simulink model "TBRe19_ECU_1_WORKING_190718"  (R2017b)
settings: Solver=FixedStepDiscrete  StartTime=0.0  StopTime=inf  FixedStep=0.0001  RelTol=1e-3
PostLoadFcn:
  | model_init();
libraries: simulink x17
(part 1 of 6)
settings Model: SimulationMode=external  Creator=agf25  LastModifiedBy=Peter
settings DataIOCC: LimitDataPoints=on
settings OptimizationCC: DefaultParameterBehavior=Inlined  EfficientFloat2IntCast=on  LifeSpan=inf
settings DebuggingCC: AllowSymbolicDim=off  SFUnexpectedBacktrackingDiag=warning  SFNoUnconditionalDefaultTransitionDiag=warning  SFExecutionAtInitializationDiag=none
settings ModelReferenceCC: PropagateSignalLabelsOutOfModel=off
settings RTWCC: SystemTargetFile=nsi_mpc.tlc  MakeCommand=nsi_make  TemplateMakefile=nsi_mpc.tmf  Description=RTW Coder for MUXLAB4
settings CodeAppCC: StateflowObjectComments=on
settings STFCustomTargetCC: MATLABClassNameForMDSCustomization=Simulink.SoftwareTarget.TargetSpecificTriggerConfigurationBase  SystemTargetFile=nsi_mpc.tlc
settings ConfigComp: CovMetricSettings=dw  CovHtmlReporting=on  CovSaveCumulativeToWorkspaceVar=on  CovSaveSingleToWorkspaceVar=on  CovExternalEMLEnable=off
settings SimscapeCC: SimscapeNormalizeSystem=off
settings ConfigurationSet: Description=SimMechanics 2G

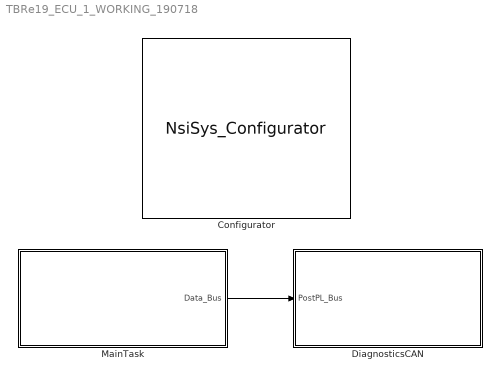
== system TBRe19_ECU_1_WORKING_190718 ==
  Configurator : S-Function  FunctionName=NsiSys_Configurator  Parameters=main,io,nbof_can,can,ccp,flash,nbof_lin,lin,tasks  SFunctionDeploymentMode=off  EnableBusSupport=off  mask(Configurator block){main=Config description;01/01/2011;0;0.000000, io=2.5;0;1;1;1;1;1;1;1, nbof_can=5, can=1;HIGH_SPEED;500Kbps;No;C:\Users\Peter\Google_Drive\Year_5\TBRe\03-Design_Files\ECU\ECU-Model\TBRe19_DBC.dbc;0;1;1Mbits;0;HIGH_SPEED;500Kbps;120 Ohm;C:\Users\TBRe-admin\Documents\Database\TBRe19_DBC_190517.dbc;0;0;1Mbits;0;HIGH_SPEED;1000Kbps;120 Ohm;D:\TOOLS\MUXLINK\R2011b\MUXlink\misc\BASE_CAN_MUXLAB4.dbc;0;0;1Mbits;0;HIGH_SPEED;500Kbps;120 Ohm;D:\TOOLS\MUXLINK\R2011b\MUXlink\misc\j1939_adapt.dbc;0;1;1Mbits;0;HIGH_SPEED;1000Kbps;No;D:\TOOLS\MUXLINK\R2011b\MUXlink\misc\BASE_CAN_MUXLAB4.dbc;0;0;1Mbits, ccp=2;0x100;0x200;0;0;0x0;0x0;0;0x13, flash=Gearing_Ratio;No;Unsigned Byte;3;1;Wheel_Size;No;Unsigned Byte;450;1;Brake1_High;No;Unsigned Word;900;1;Brake2_High;No;Unsigned Word;900;1;Throttle1_High;No;Unsigned Word;4800;1;Throttle2_High;No;Unsigned Word;4200;1;Brake1_Low;No;Unsigned Word;500;1;Brake2_Low;No;Unsigned Word;500;1;Throttle1_Low;No;Unsigned Word;904;1;Throttle2_Low;No;Unsigned Word;290;1;Max_Torque_Std;No;Unsigned Byte;140;1;Max_Torque_Boost;No;Unsigned Byte;240;1;MCU_Ignition;No;Boolean;1;1;LV_Low_Voltage_Warning;No;Unsigned Word;25000;1;MCUMotor_Temp_Warning;No;Unsigned Word;60;1;Target_Slip_Ratio;No;Single Float;0.15;1;TC_P_Gain;No;Unsigned Byte;1000;1;MinTC_Torque;No;Unsigned Byte;20;1;Max_Regen;No;Unsigned Byte;30;1;Throttle_Active_Threshold;No;Unsigned Byte;5;1;Brake_Active_Threshold;No;Unsigned Byte;15;1;INV_Torque_limit;No;Signed Word;210;1;INV_Speed_Limit_Fwd;No;Signed Word;3000;1;INV_Speed_limit_Rev;No;Signed Word;-3000;1;INV_DC_Link_Target;No;Signed Word;60;1;INV_DC_Link_Regen_Imax;No;Signed Word;-10;1;INV_DC_Link_Discharge_Imax;No;Signed Word;200;1;INV_Regen_Torque_Limit;No;Signed Word;-10;1;INV_Id_Debug;No;Signed Word;0;1;INV_Iq_debug;No;Signed Word;0;1, nbof_lin=2, lin=0;D:\TOOLS\MUXLINK\R2011b\MUXlink\misc\lindb.ldf;1;0.0;0.0;0.000;0.000;0.000000;0,0;0;D:\TOOLS\MUXLINK\R2011b\MUXlink\misc\lindb.ldf;1;0.0;0.0;0.000;0.000;0.000000;0,0, tasks=DiagnosticsCAN;[0.1];MainTask;[0.01]}
      mask prompts: nbof_can "nbof can"
      mask help: This block permits to set general parameters to use a MUXlink model
      mask init:
      | NsiSys_Configurator_InitializationFcn();
      settings: OpenFcn=NsiSys_Configurator_OpenFcn();
      mask Help:
      | eval('block=get_param(gcb, ''RTWdata'');')
      | web([docroot '\toolbox\MUXlink\html\blocks/' block.MUXlink_BlockType '.html'])
      mask Callback main: NsiSys_Configurator_ApplyFcn(1);
      mask Callback io: NsiSys_Configurator_ApplyFcn(2);
      mask Callback nbof_can: NsiSys_Configurator_ApplyFcn(3);
      mask Callback can: NsiSys_Configurator_ApplyFcn(4);
      mask Callback ccp: NsiSys_Configurator_ApplyFcn(5);
      mask Callback flash: NsiSys_Configurator_ApplyFcn(6);
      mask Callback nbof_lin: NsiSys_Configurator_ApplyFcn(7);
      mask Callback lin: NsiSys_Configurator_ApplyFcn(8);
      mask Callback tasks: NsiSys_Configurator_ApplyFcn(9);
      mask Display: image(imread('MUXLAB4.bmp'));text(0.5, 0.2, '', 'horizontalAlignment', 'center', 'verticalAlignment', 'base');
  DiagnosticsCAN : Subsystem  TreatAsAtomicUnit=on  SystemSampleTime=[0.1]  RTWFcnName=DiagnosticsCAN  RTWFileName=FileTaskFcn
      mask init:
      | NsiSys_SubSystemTask_InitializationFcn();
      settings: OpenFcn=NsiSys_SubSystemTask_OpenFcn();  RTWSystemCode=Nonreusable function  RTWFcnNameOpts=User specified  RTWFileNameOpts=Use function name
      mask Display: image(imread('nsi.bmp'));text(0.45, 0.9, 'task()');plot([0.05 0.05 0.05 0.05 0.05 0.05 0.05 0.05 0.05 0.05]);fprintf('DiagnosticsCAN\n/ 100.0ms / 10.0ms /\nEvent');
  MainTask : Subsystem  TreatAsAtomicUnit=on  SystemSampleTime=[0.01]  RTWFcnName=MainTask  RTWFileName=FileTaskFcn
      mask init:
      | NsiSys_SubSystemTask_InitializationFcn();
      settings: OpenFcn=NsiSys_SubSystemTask_OpenFcn();  RTWSystemCode=Nonreusable function  RTWFcnNameOpts=User specified  RTWFileNameOpts=Use function name
      mask Display: image(imread('nsi.bmp'));text(0.45, 0.9, 'task()');plot([0.05 0.05 0.05 0.05 0.05 0.05 0.05 0.05 0.05 0.05]);fprintf('MainTask\n/ 10.0ms / 0.0ms /\nEvent');
  wires:
  MainTask/1(Data_Bus) -> DiagnosticsCAN/1(PostPL_Bus)

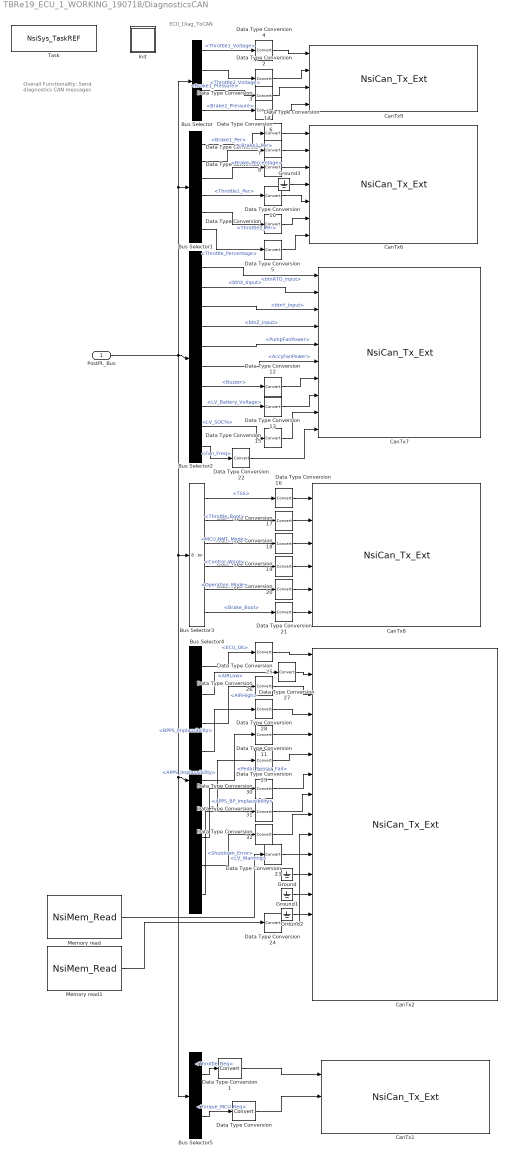
== system TBRe19_ECU_1_WORKING_190718/DiagnosticsCAN ==
  note: ECU_Diag_ToCAN
  note: Overall Functionality:
      | Send diagnostics CAN messages
  PostPL_Bus : Inport
  Bus Selector : BusSelector  OutputSignals=VFL_Data.PrePL_Data.DAL_Data.DAL_Hardwired.Throttle1_Voltage,VFL_Data.PrePL_Data.DAL_Data.DAL_Hardwired.Throttle2_Voltage,VFL_Data.PrePL_Data.DAL_Data.DAL_Hardwired.Brake1_Pressure,VFL_Data.PrePL_Data.DAL_Data.DAL_Hardwired.Brake2_Pressure
  Bus Selector1 : BusSelector  OutputSignals=VFL_Data.PrePL_Data.Pedal_Box_Data.Brake1_Per,VFL_Data.PrePL_Data.Pedal_Box_Data.Brake2_Per,VFL_Data.PrePL_Data.Pedal_Box_Data.Brake_Percentage,VFL_Data.PrePL_Data.Pedal_Box_Data.Throttle1_Per,VFL_Data.PrePL_Data.Pedal_Box_Data.Throttle2_Per,VFL_Data.PrePL_Data.Pedal_Box_Data.Throttle_Percentage
  Bus Selector2 : BusSelector  OutputSignals=VFL_Data.PrePL_Data.DAL_Data.DAL_Hardwired.btnRTD_Input,VFL_Data.PrePL_Data.DAL_Data.DAL_Hardwired.btnX_Input,VFL_Data.PrePL_Data.DAL_Data.DAL_Hardwired.btnY_Input,VFL_Data.PrePL_Data.DAL_Data.DAL_Hardwired.btnZ_Input,Hardwired_Peripherals.PumpFanPower,Hardwired_Peripherals.AccyFanPower,Hardwired_Peripherals.Buzzer,VFL_Data.PrePL_Data.LV_Battery.LV_Battery_Voltage,VFL_Data.PrePL_Data.LV_Battery.LV_SOC%,VFL_Data.PrePL_Data.DAL_Data.DAL_Hardwired.Fan_Freq
  Bus Selector3 : BusSelector  OutputSignals=VFL_Data.VOM_Data.TSS,VFL_Data.PrePL_Data.Pedal_Box_Data.Throttle_Bool,VFL_Data.VOM_Data.MCU_NMT_Mode,VFL_Data.VOM_Data.Control_Word,VFL_Data.VOM_Data.Operation_Mode,VFL_Data.PrePL_Data.Pedal_Box_Data.Brake_Bool
  Bus Selector4 : BusSelector  OutputSignals=Hardwired_Peripherals.ECU_Ok,VFL_Data.PrePL_Data.DAL_Data.DAL_Hardwired.AIRLow,VFL_Data.PrePL_Data.DAL_Data.DAL_Hardwired.AIRHigh,VFL_Data.PrePL_Data.Pedal_Box_Data.BPPS_Implausibility,VFL_Data.PrePL_Data.Pedal_Box_Data.Pedal_Sensor_Fail,VFL_Data.PrePL_Data.Pedal_Box_Data.APPS_Implausibility,VFL_Data.PrePL_Data.Pedal_Box_Data.APPS_BP_Implausibility,VFL_Data.PrePL_Data.LV_Battery.LV_Warning,VFL_Data.PrePL_Data.DAL_Data.DAL_CAN.DAL_SENSORCAN.Shutdown_Error
  Bus Selector5 : BusSelector  OutputSignals=VFL_Data.Drive_Data.Throttle_Req,VFL_Data.Drive_Data.Torque_MCU_Req
  CanTx1 : S-Function  FunctionName=NsiCan_Tx_Ext  Parameters=data_can,channel,msg_name,ident,ident_type,dlc,signals,is_physical,is_canfd,is_crc  SFunctionDeploymentMode=off  EnableBusSupport=off  mask(MUXlink Can Tx){data_can=1;HIGH_SPEED;500Kbps;No;C:\Users\TBRe-admin\Documents\TBReVCU\TBRe19_DBC.dbc;0;;;0;HIGH_SPEED;500Kbps;120 Ohm;C:\Users\TBRe-admin\Documents\Database\TBRe19_DBC_190517.dbc;0;;;0;HIGH_SPEED;1000Kbps;120 Ohm;D:\TOOLS\MUXLINK\R2011b\MUXlink\misc\BASE_CAN_MUXLAB4.dbc;0;;;0;HIGH_SPEED;500Kbps;120 Ohm;D:\TOOLS\MUXLINK\R2011b\MUXlink\misc\j1939_adapt.dbc;0;;;0;HIGH_SPEED;1000Kbps;No;D:\TOOLS\MUXLINK\R2011b\MUXlink\misc\BASE_CAN_MUXLAB4.dbc;0;;, channel=1, msg_name=VCU_Torque, ident=0x706, ident_type=STD, dlc=5, signals=ECU_TorqueReq;1;0;-16;0.100000;0.000000;Percent;ECU_TorqueAcut;1;16;-16;0.100000;0.000000;Percent;Max_Torque;1;32;-8;1.000000;0.000000;_, is_physical=1, is_canfd=0, is_crc=0}
      mask prompts: data_can "data can"; msg_name "msg name"
      mask help: Transmit a frame on a CAN Channel.
      mask init:
      | NsiCan_Tx_Ext_InitializationFcn();
      settings: OpenFcn=NsiCan_Tx_Ext_OpenFcn();
      mask Help:
      | eval('block=get_param(gcb, ''RTWdata'');')
      | web([docroot '\toolbox\MUXlink\html\blocks/' block.MUXlink_BlockType '.html'])
      mask Callback data_can: NsiCan_Tx_Ext_ApplyFcn(1);
      mask Callback channel: NsiCan_Tx_Ext_ApplyFcn(2);
      mask Callback msg_name: NsiCan_Tx_Ext_ApplyFcn(3);
      mask Callback ident: NsiCan_Tx_Ext_ApplyFcn(4);
      mask Callback ident_type: NsiCan_Tx_Ext_ApplyFcn(5);
      mask Callback dlc: NsiCan_Tx_Ext_ApplyFcn(6);
      mask Callback signals: NsiCan_Tx_Ext_ApplyFcn(7);
      mask Callback is_physical: NsiCan_Tx_Ext_ApplyFcn(7);
      mask Callback is_canfd: NsiCan_Tx_Ext_ApplyFcn(7);
      mask Callback is_crc: NsiCan_Tx_Ext_ApplyFcn(7);
      mask Display: image(imread('nsi.bmp'));text(0.5, 0.1, 'TX_VCU_Torque_CAN1', 'horizontalAlignment', 'center', 'verticalAlignment', 'base');plot([0.05 0.05 0.05 0.05 0.05 0.05 0.05 0.05 0.05 0.05]); port_label('input',1, 'ECU_TorqueReq'); port_label('input',2, 'ECU_TorqueAcut'); port_label('input',3, 'Max_Torque');
  CanTx2 : S-Function  FunctionName=NsiCan_Tx_Ext  Parameters=data_can,channel,msg_name,ident,ident_type,dlc,signals,is_physical,is_canfd,is_crc  SFunctionDeploymentMode=off  EnableBusSupport=off  mask(MUXlink Can Tx){data_can=1;HIGH_SPEED;500Kbps;No;C:\Users\TBRe-admin\Documents\TBReVCU\TBRe19_DBC.dbc;0;;;0;HIGH_SPEED;500Kbps;120 Ohm;C:\Users\TBRe-admin\Documents\Database\TBRe19_DBC_190517.dbc;0;;;0;HIGH_SPEED;1000Kbps;120 Ohm;D:\TOOLS\MUXLINK\R2011b\MUXlink\misc\BASE_CAN_MUXLAB4.dbc;0;;;0;HIGH_SPEED;500Kbps;120 Ohm;D:\TOOLS\MUXLINK\R2011b\MUXlink\misc\j1939_adapt.dbc;0;;;0;HIGH_SPEED;1000Kbps;No;D:\TOOLS\MUXLINK\R2011b\MUXlink\misc\BASE_CAN_MUXLAB4.dbc;0;;, channel=1, msg_name=VCU_Diagnostics, ident=0x700, ident_type=STD, dlc=4, signals=Shutdown_ECU;1;22;-1;1.000000;0.000000;_;Low_AIR_Status;1;20;-1;1.000000;0.000000;_;High_AIR_Status;1;21;1;1.000000;0.000000;_;BPPS_Implausibility;1;16;-1;1.000000;0.000000;_;Pedal_Sensor_Fail;1;24;8;1.000000;0.000000;_;APPS_Implausibility;1;17;1;1.000000;0.000000;_;APPS_BP_Implausibility;1;18;1;1.000000;0.000000;_;Shutdown_CarShutdown;1;23;1;1.000000;0.000000;_;LV_Battery_Warning;1;19;1;1.000000;0.000000;_;GearingRatio;1;8;8;0.100000;0.000000;_;Wheel_Size;1;0;8;0.100000;0.000000;m;Boost_on;1;34;-1;1.000000;0.000000;_;TC_on;1;33;-1;1.000000;0.000000;_;RegenBool;1;32;-1;1.000000;0.000000;_;VCU_Day;1;35;5;1.000000;0.000000;_;VCU_Month;1;40;8;1.000000;0.000000;_;VCU_Version;1;56;8;1.000000;0.000000;_;VCU_Year;1;48;8;1.000000;0.000000;_, is_physical=1, is_canfd=0, is_crc=0}
      mask prompts: data_can "data can"; msg_name "msg name"
      mask help: Transmit a frame on a CAN Channel.
      mask init:
      | NsiCan_Tx_Ext_InitializationFcn();
      settings: OpenFcn=NsiCan_Tx_Ext_OpenFcn();
      mask Help:
      | eval('block=get_param(gcb, ''RTWdata'');')
      | web([docroot '\toolbox\MUXlink\html\blocks/' block.MUXlink_BlockType '.html'])
      mask Callback data_can: NsiCan_Tx_Ext_ApplyFcn(1);
      mask Callback channel: NsiCan_Tx_Ext_ApplyFcn(2);
      mask Callback msg_name: NsiCan_Tx_Ext_ApplyFcn(3);
      mask Callback ident: NsiCan_Tx_Ext_ApplyFcn(4);
      mask Callback ident_type: NsiCan_Tx_Ext_ApplyFcn(5);
      mask Callback dlc: NsiCan_Tx_Ext_ApplyFcn(6);
      mask Callback signals: NsiCan_Tx_Ext_ApplyFcn(7);
      mask Callback is_physical: NsiCan_Tx_Ext_ApplyFcn(7);
      mask Callback is_canfd: NsiCan_Tx_Ext_ApplyFcn(7);
      mask Callback is_crc: NsiCan_Tx_Ext_ApplyFcn(7);
      mask Display: image(imread('nsi.bmp'));text(0.5, 0.3, 'TX_VCU_Diagnostics_CAN1', 'horizontalAlignment', 'center', 'verticalAlignment', 'base');plot([0.05 0.05 0.05 0.05 0.05 0.05 0.05 0.05 0.05 0.05]); port_label('input',1, 'Shutdown_ECU'); port_label('input',2, 'Low_AIR_Status'); port_label('input',3, 'High_AIR_Status'); port_label('input',4, 'BPPS_Implausibility'); port_label('input',5, 'Pedal_Sensor_Fail'); port_label('input',6, 'APPS_Implausibility'); port_label('input',7, 'APPS_BP_Implausibility'); port_label('input',8, 'Shutdown_CarShutdown'); port_label('input',9, 'LV_Battery_Warning'); port_label('input',10, 'GearingRatio'); port_label('input',11, 'Wheel_Size'); port_label('input',12, 'Boost_on'); port_label('input',13, 'TC_on'); port_label('input',14, 'RegenBool'); port_label('input',15, 'VCU_Day'); port_label('input',16, 'VCU_Month'); port_label('input',17, 'VCU_Version'); port_label('input',18, 'VCU_Year');
  CanTx6 : S-Function  FunctionName=NsiCan_Tx_Ext  Parameters=data_can,channel,msg_name,ident,ident_type,dlc,signals,is_physical,is_canfd,is_crc  SFunctionDeploymentMode=off  EnableBusSupport=off  mask(MUXlink Can Tx){data_can=1;HIGH_SPEED;500Kbps;No;C:\Users\TBRe-admin\Documents\TBReVCU\TBRe19_DBC.dbc;0;;;0;HIGH_SPEED;500Kbps;120 Ohm;C:\Users\TBRe-admin\Documents\Database\TBRe19_DBC_190517.dbc;0;;;0;HIGH_SPEED;1000Kbps;120 Ohm;D:\TOOLS\MUXLINK\R2011b\MUXlink\misc\BASE_CAN_MUXLAB4.dbc;0;;;0;HIGH_SPEED;500Kbps;120 Ohm;D:\TOOLS\MUXLINK\R2011b\MUXlink\misc\j1939_adapt.dbc;0;;;0;HIGH_SPEED;1000Kbps;No;D:\TOOLS\MUXLINK\R2011b\MUXlink\misc\BASE_CAN_MUXLAB4.dbc;0;;, channel=1, msg_name=VCU_Pedal_Percentages, ident=0x702, ident_type=STD, dlc=7, signals=Brake1_Percentage;1;24;8;1.000000;0.000000;%;Brake2_Percentage;1;32;8;1.000000;0.000000;%;Brake_Percentage;1;48;8;1.000000;0.000000;%;BrakePot_Percentage;1;40;8;1.000000;0.000000;%;Throttle1_Percent;1;0;8;1.000000;0.000000;%;Throttle2_Percentage;1;8;8;1.000000;0.000000;%;Throttle_Percentage;1;16;8;1.000000;0.000000;%, is_physical=1, is_canfd=0, is_crc=0}
      mask prompts: data_can "data can"; msg_name "msg name"
      mask help: Transmit a frame on a CAN Channel.
      mask init:
      | NsiCan_Tx_Ext_InitializationFcn();
      settings: OpenFcn=NsiCan_Tx_Ext_OpenFcn();
      mask Help:
      | eval('block=get_param(gcb, ''RTWdata'');')
      | web([docroot '\toolbox\MUXlink\html\blocks/' block.MUXlink_BlockType '.html'])
      mask Callback data_can: NsiCan_Tx_Ext_ApplyFcn(1);
      mask Callback channel: NsiCan_Tx_Ext_ApplyFcn(2);
      mask Callback msg_name: NsiCan_Tx_Ext_ApplyFcn(3);
      mask Callback ident: NsiCan_Tx_Ext_ApplyFcn(4);
      mask Callback ident_type: NsiCan_Tx_Ext_ApplyFcn(5);
      mask Callback dlc: NsiCan_Tx_Ext_ApplyFcn(6);
      mask Callback signals: NsiCan_Tx_Ext_ApplyFcn(7);
      mask Callback is_physical: NsiCan_Tx_Ext_ApplyFcn(7);
      mask Callback is_canfd: NsiCan_Tx_Ext_ApplyFcn(7);
      mask Callback is_crc: NsiCan_Tx_Ext_ApplyFcn(7);
      mask Display: image(imread('nsi.bmp'));text(0.5, 0.1, 'TX_VCU_Pedal_Percentages_CAN1', 'horizontalAlignment', 'center', 'verticalAlignment', 'base');plot([0.05 0.05 0.05 0.05 0.05 0.05 0.05 0.05 0.05 0.05]); port_label('input',1, 'Brake1_Percentage'); port_label('input',2, 'Brake2_Percentage'); port_label('input',3, 'Brake_Percentage'); port_label('input',4, 'BrakePot_Percentage'); port_label('input',5, 'Throttle1_Percent'); port_label('input',6, 'Throttle2_Percentage'); port_label('input',7, 'Throttle_Percentage');
  CanTx7 : S-Function  FunctionName=NsiCan_Tx_Ext  Parameters=data_can,channel,msg_name,ident,ident_type,dlc,signals,is_physical,is_canfd,is_crc  SFunctionDeploymentMode=off  EnableBusSupport=off  mask(MUXlink Can Tx){data_can=1;HIGH_SPEED;500Kbps;No;C:\Users\TBRe-admin\Documents\TBReVCU\TBRe19_DBC.dbc;0;;;0;HIGH_SPEED;500Kbps;120 Ohm;C:\Users\TBRe-admin\Documents\Database\TBRe19_DBC_190517.dbc;0;;;0;HIGH_SPEED;1000Kbps;120 Ohm;D:\TOOLS\MUXLINK\R2011b\MUXlink\misc\BASE_CAN_MUXLAB4.dbc;0;;;0;HIGH_SPEED;500Kbps;120 Ohm;D:\TOOLS\MUXLINK\R2011b\MUXlink\misc\j1939_adapt.dbc;0;;;0;HIGH_SPEED;1000Kbps;No;D:\TOOLS\MUXLINK\R2011b\MUXlink\misc\BASE_CAN_MUXLAB4.dbc;0;;, channel=1, msg_name=VCU_HW_IO, ident=0x701, ident_type=STD, dlc=4, signals=Console_RTD;1;0;1;1.000000;0.000000;Bool;Console_X;1;3;1;1.000000;0.000000;Bool;Consle_Y;1;2;-1;1.000000;0.000000;Bool;Console_Z;1;1;-1;1.000000;0.000000;_;Coolant_Pump_Fan;1;5;1;1.000000;0.000000;_;Coolant_AccyFan;1;6;-1;1.000000;0.000000;_;Buzzer;1;7;1;1.000000;0.000000;_;LV_Battery_Voltage;1;16;16;1.000000;0.000000;mV;LV_Battery_SOC;1;8;8;1.000000;0.000000;_;AccyFanFreq;1;32;8;1.000000;0.000000;Hz, is_physical=1, is_canfd=0, is_crc=0}
      mask prompts: data_can "data can"; msg_name "msg name"
      mask help: Transmit a frame on a CAN Channel.
      mask init:
      | NsiCan_Tx_Ext_InitializationFcn();
      settings: OpenFcn=NsiCan_Tx_Ext_OpenFcn();
      mask Help:
      | eval('block=get_param(gcb, ''RTWdata'');')
      | web([docroot '\toolbox\MUXlink\html\blocks/' block.MUXlink_BlockType '.html'])
      mask Callback data_can: NsiCan_Tx_Ext_ApplyFcn(1);
      mask Callback channel: NsiCan_Tx_Ext_ApplyFcn(2);
      mask Callback msg_name: NsiCan_Tx_Ext_ApplyFcn(3);
      mask Callback ident: NsiCan_Tx_Ext_ApplyFcn(4);
      mask Callback ident_type: NsiCan_Tx_Ext_ApplyFcn(5);
      mask Callback dlc: NsiCan_Tx_Ext_ApplyFcn(6);
      mask Callback signals: NsiCan_Tx_Ext_ApplyFcn(7);
      mask Callback is_physical: NsiCan_Tx_Ext_ApplyFcn(7);
      mask Callback is_canfd: NsiCan_Tx_Ext_ApplyFcn(7);
      mask Callback is_crc: NsiCan_Tx_Ext_ApplyFcn(7);
      mask Display: image(imread('nsi.bmp'));text(0.5, 0.3, 'TX_VCU_HW_IO_CAN1', 'horizontalAlignment', 'center', 'verticalAlignment', 'base');plot([0.05 0.05 0.05 0.05 0.05 0.05 0.05 0.05 0.05 0.05]); port_label('input',1, 'Console_RTD'); port_label('input',2, 'Console_X'); port_label('input',3, 'Consle_Y'); port_label('input',4, 'Console_Z'); port_label('input',5, 'Coolant_Pump_Fan'); port_label('input',6, 'Coolant_AccyFan'); port_label('input',7, 'Buzzer'); port_label('input',8, 'LV_Battery_Voltage'); port_label('input',9, 'LV_Battery_SOC'); port_label('input',10, 'AccyFanFreq');
  CanTx8 : S-Function  FunctionName=NsiCan_Tx_Ext  Parameters=data_can,channel,msg_name,ident,ident_type,dlc,signals,is_physical,is_canfd,is_crc  SFunctionDeploymentMode=off  EnableBusSupport=off  mask(MUXlink Can Tx){data_can=1;HIGH_SPEED;500Kbps;No;C:\Users\TBRe-admin\Documents\TBReVCU\TBRe19_DBC.dbc;0;;;0;HIGH_SPEED;500Kbps;120 Ohm;C:\Users\TBRe-admin\Documents\Database\TBRe19_DBC_190517.dbc;0;;;0;HIGH_SPEED;1000Kbps;120 Ohm;D:\TOOLS\MUXLINK\R2011b\MUXlink\misc\BASE_CAN_MUXLAB4.dbc;0;;;0;HIGH_SPEED;500Kbps;120 Ohm;D:\TOOLS\MUXLINK\R2011b\MUXlink\misc\j1939_adapt.dbc;0;;;0;HIGH_SPEED;1000Kbps;No;D:\TOOLS\MUXLINK\R2011b\MUXlink\misc\BASE_CAN_MUXLAB4.dbc;0;;, channel=1, msg_name=VCU_Vehicle_Functionality, ident=0x704, ident_type=STD, dlc=4, signals=Tractive_System_Startup;1;24;1;1.000000;0.000000;_;Throttle_Bool;1;25;1;1.000000;0.000000;_;MCU_NMT_Mode;1;16;8;1.000000;0.000000;_;Control_Word;1;0;8;1.000000;0.000000;_;Vehicle_Operation;1;8;8;1.000000;0.000000;_;Brake_Bool;1;26;1;1.000000;0.000000;_, is_physical=1, is_canfd=0, is_crc=0}
      mask prompts: data_can "data can"; msg_name "msg name"
      mask help: Transmit a frame on a CAN Channel.
      mask init:
      | NsiCan_Tx_Ext_InitializationFcn();
      settings: OpenFcn=NsiCan_Tx_Ext_OpenFcn();
      mask Help:
      | eval('block=get_param(gcb, ''RTWdata'');')
      | web([docroot '\toolbox\MUXlink\html\blocks/' block.MUXlink_BlockType '.html'])
      mask Callback data_can: NsiCan_Tx_Ext_ApplyFcn(1);
      mask Callback channel: NsiCan_Tx_Ext_ApplyFcn(2);
      mask Callback msg_name: NsiCan_Tx_Ext_ApplyFcn(3);
      mask Callback ident: NsiCan_Tx_Ext_ApplyFcn(4);
      mask Callback ident_type: NsiCan_Tx_Ext_ApplyFcn(5);
      mask Callback dlc: NsiCan_Tx_Ext_ApplyFcn(6);
      mask Callback signals: NsiCan_Tx_Ext_ApplyFcn(7);
      mask Callback is_physical: NsiCan_Tx_Ext_ApplyFcn(7);
      mask Callback is_canfd: NsiCan_Tx_Ext_ApplyFcn(7);
      mask Callback is_crc: NsiCan_Tx_Ext_ApplyFcn(7);
      mask Display: image(imread('nsi.bmp'));text(0.5, 0.3, 'TX_VCU_Vehicle_Functionality_CAN1', 'horizontalAlignment', 'center', 'verticalAlignment', 'base');plot([0.05 0.05 0.05 0.05 0.05 0.05 0.05 0.05 0.05 0.05]); port_label('input',1, 'Tractive_System_Startup'); port_label('input',2, 'Throttle_Bool'); port_label('input',3, 'MCU_NMT_Mode'); port_label('input',4, 'Control_Word'); port_label('input',5, 'Vehicle_Operation'); port_label('input',6, 'Brake_Bool');
  CanTx9 : S-Function  FunctionName=NsiCan_Tx_Ext  Parameters=data_can,channel,msg_name,ident,ident_type,dlc,signals,is_physical,is_canfd,is_crc  SFunctionDeploymentMode=off  EnableBusSupport=off  mask(MUXlink Can Tx){data_can=1;HIGH_SPEED;500Kbps;No;C:\Users\TBRe-admin\Documents\Database\TBRe19_DBC_190621.dbc;0;;;0;HIGH_SPEED;500Kbps;120 Ohm;C:\Users\TBRe-admin\Documents\Database\TBRe19_DBC_190517.dbc;0;;;0;HIGH_SPEED;1000Kbps;120 Ohm;D:\TOOLS\MUXLINK\R2011b\MUXlink\misc\BASE_CAN_MUXLAB4.dbc;0;;;0;HIGH_SPEED;500Kbps;120 Ohm;D:\TOOLS\MUXLINK\R2011b\MUXlink\misc\j1939_adapt.dbc;0;;;0;HIGH_SPEED;1000Kbps;No;D:\TOOLS\MUXLINK\R2011b\MUXlink\misc\BASE_CAN_MUXLAB4.dbc;0;;, channel=1, msg_name=VCU_Pedal_Voltages, ident=0x703, ident_type=STD, dlc=8, signals=Throttle1_Voltage;1;0;16;1.000000;0.000000;mV;Throttle2_Voltage;1;32;16;1.000000;0.000000;mV;Brake1_Voltage;1;16;16;1.000000;0.000000;mV;Brake2_Voltage;1;48;16;1.000000;0.000000;mV, is_physical=0, is_canfd=0, is_crc=0}
      mask prompts: data_can "data can"; msg_name "msg name"
      mask help: Transmit a frame on a CAN Channel.
      mask init:
      | NsiCan_Tx_Ext_InitializationFcn();
      settings: OpenFcn=NsiCan_Tx_Ext_OpenFcn();
      mask Help:
      | eval('block=get_param(gcb, ''RTWdata'');')
      | web([docroot '\toolbox\MUXlink\html\blocks/' block.MUXlink_BlockType '.html'])
      mask Callback data_can: NsiCan_Tx_Ext_ApplyFcn(1);
      mask Callback channel: NsiCan_Tx_Ext_ApplyFcn(2);
      mask Callback msg_name: NsiCan_Tx_Ext_ApplyFcn(3);
      mask Callback ident: NsiCan_Tx_Ext_ApplyFcn(4);
      mask Callback ident_type: NsiCan_Tx_Ext_ApplyFcn(5);
      mask Callback dlc: NsiCan_Tx_Ext_ApplyFcn(6);
      mask Callback signals: NsiCan_Tx_Ext_ApplyFcn(7);
      mask Callback is_physical: NsiCan_Tx_Ext_ApplyFcn(7);
      mask Callback is_canfd: NsiCan_Tx_Ext_ApplyFcn(7);
      mask Callback is_crc: NsiCan_Tx_Ext_ApplyFcn(7);
      mask Display: image(imread('nsi.bmp'));text(0.5, 0.3, 'TX_VCU_Pedal_Voltages_CAN1', 'horizontalAlignment', 'center', 'verticalAlignment', 'base');plot([0.05 0.05 0.05 0.05 0.05 0.05 0.05 0.05 0.05 0.05]); port_label('input',1, 'Throttle1_Voltage'); port_label('input',2, 'Throttle2_Voltage'); port_label('input',3, 'Brake1_Voltage'); port_label('input',4, 'Brake2_Voltage');
  Data Type Conversion{,1..32} (33 alike) : DataTypeConversion
  Ground{,1..3} (4 alike) : Ground
  Init : Subsystem  mask(System Initialize){}
      mask help: Add code to a systems Initialize function
      settings: CopyFcn=cccopyfcn(gcb)  OpenFcn=ccopenfcn('System Initialize Function')
      mask Help: This block contains text fields to insert custom user code sections at the declaration, execution and exit sections of the systems initialize function.  By placing this block inside a subsytem, the custom user code will appear in that subsystems function.
      mask Display: disp('I()')
  Memory read : S-Function  FunctionName=NsiMem_Read  Parameters=name_var,type_var,size_var,tunable_var  SFunctionDeploymentMode=off  EnableBusSupport=off  mask(Memory read){name_var=Wheel_Size, type_var=Unsigned Byte, size_var=1, tunable_var=on}
      mask prompts: name_var "Variable name :"; type_var "Type :"; size_var "Dim of table :"; tunable_var "Is Tunable By USB?"
      mask help: Reads current value of variable memory declared in the configurator block in calibration page.
      mask init:
      | NsiMem_Read_InitializationFcn();
      settings: OpenFcn=NsiMem_Read_OpenFcn();
      mask Help:
      | eval('block=get_param(gcb, ''RTWdata'');')
      | web([docroot '\toolbox\MUXlink\html\blocks/' block.MUXlink_BlockType '.html'])
      mask TypeOptions name_var: Gearing_Ratio | Wheel_Size | Brake1_High | Brake2_High | Throttle1_High | Throttle2_High | Brake1_Low | Brake2_Low | Throttle1_Low | Throttle2_Low | Max_Torque_Std | Max_Torque_Boost | MCU_Ignition | LV_Low_Voltage_Warning | MCUMotor_Temp_Warning | Target_Slip_Ratio | TC_P_Gain | MinTC_Torque | Max_Regen | Throttle_Active_Threshold | Brake_Active_Threshold | INV_Torque_limit | INV_Speed_Limit_Fwd | INV_Speed_limit_Rev | INV_DC_Link_Target | INV_DC_Link_Regen_Imax | INV_DC_Link_Discharge_Imax | INV_Regen_Torque_Limit | INV_Id_Debug | INV_Iq_debug
      mask Callback name_var: NsiMem_Read_ApplyFcn(1);
      mask TypeOptions type_var: Boolean | Signed Byte | Unsigned Byte | Signed Word | Unsigned Word | Signed Double Word | Unsigned Double Word | Single Float | Double Float
      mask Callback type_var: NsiMem_Read_ApplyFcn(2);
      mask Callback size_var: NsiMem_Read_ApplyFcn(3);
      mask Callback tunable_var: NsiMem_Read_ApplyFcn(4);
      mask Display: image(imread('nsi.bmp'));text(0.5, 0.35, 'Wheel_Size', 'horizontalAlignment', 'center', 'verticalAlignment', 'base');plot([0.05 0.05 0.05 0.05 0.05 0.05 0.05 0.05 0.05 0.05]);port_label('output', 1, 'Read');
  Memory read1 : S-Function  FunctionName=NsiMem_Read  Parameters=name_var,type_var,size_var,tunable_var  SFunctionDeploymentMode=off  EnableBusSupport=off  mask(Memory read){name_var=Gearing_Ratio, type_var=Unsigned Byte, size_var=1, tunable_var=on}
      mask prompts: name_var "Variable name :"; type_var "Type :"; size_var "Dim of table :"; tunable_var "Is Tunable By USB?"
      mask help: Reads current value of variable memory declared in the configurator block in calibration page.
      mask init:
      | NsiMem_Read_InitializationFcn();
      settings: OpenFcn=NsiMem_Read_OpenFcn();
      mask Help:
      | eval('block=get_param(gcb, ''RTWdata'');')
      | web([docroot '\toolbox\MUXlink\html\blocks/' block.MUXlink_BlockType '.html'])
      mask TypeOptions name_var: Gearing_Ratio | Wheel_Size | Brake1_High | Brake2_High | Throttle1_High | Throttle2_High | Brake1_Low | Brake2_Low | Throttle1_Low | Throttle2_Low | Max_Torque_Std | Max_Torque_Boost | MCU_Ignition | LV_Low_Voltage_Warning | MCUMotor_Temp_Warning | Target_Slip_Ratio | TC_P_Gain | MinTC_Torque | Max_Regen | Throttle_Active_Threshold | Brake_Active_Threshold | INV_Torque_limit | INV_Speed_Limit_Fwd | INV_Speed_limit_Rev | INV_DC_Link_Target | INV_DC_Link_Regen_Imax | INV_DC_Link_Discharge_Imax | INV_Regen_Torque_Limit | INV_Id_Debug | INV_Iq_debug
      mask Callback name_var: NsiMem_Read_ApplyFcn(1);
      mask TypeOptions type_var: Boolean | Signed Byte | Unsigned Byte | Signed Word | Unsigned Word | Signed Double Word | Unsigned Double Word | Single Float | Double Float
      mask Callback type_var: NsiMem_Read_ApplyFcn(2);
      mask Callback size_var: NsiMem_Read_ApplyFcn(3);
      mask Callback tunable_var: NsiMem_Read_ApplyFcn(4);
      mask Display: image(imread('nsi.bmp'));text(0.5, 0.35, 'Gearing_Ratio', 'horizontalAlignment', 'center', 'verticalAlignment', 'base');plot([0.05 0.05 0.05 0.05 0.05 0.05 0.05 0.05 0.05 0.05]);port_label('output', 1, 'Read');
  Task : S-Function  FunctionName=NsiSys_TaskREF  Parameters=task_initialised,task_periodic, task_sampletime,task_name,task_event,task_offset  SFunctionDeploymentMode=off  EnableBusSupport=off  mask(task definition){task_initialised=on, task_periodic=on, task_sampletime=[0.1], task_offset=0.01, task_name=DiagnosticsCAN, task_event=on}
      mask prompts: task_initialised "task initialised"; task_periodic "Is Periodic"; task_sampletime "Task sample time"; task_offset "Task Offset"; task_name "Task name"; task_event "Is event"
      mask help:
      | Permit to provide all parameters associated to a MUXLINK task.
      | Task can be executed periodicaly and/or on event detection.
      | If task is periodic:
      | Task sample time specify the execution period in mS [0.001   6000]
      | Task Offset specify the offset applied to the execution period
      | Task Offset < Task sample time
      mask init:
      | NsiSys_TaskREF_InitializationFcn();
      settings: OpenFcn=NsiSys_Task_OpenFcn();
      mask Callback task_initialised: NsiSys_TaskREF_ApplyFcn(1);
      mask Callback task_periodic: NsiSys_TaskREF_ApplyFcn(2);
      mask Callback task_sampletime: NsiSys_TaskREF_ApplyFcn(3);
      mask Callback task_offset: NsiSys_TaskREF_ApplyFcn(6);
      mask Callback task_name: NsiSys_TaskREF_ApplyFcn(4);
      mask Callback task_event: NsiSys_TaskREF_ApplyFcn(5);
      mask Display: text(0.5, 0.8, 't()', 'horizontalAlignment', 'center', 'verticalAlignment', 'base');text(0.5, 0.2, '/ 100.0ms / 10.0ms /', 'horizontalAlignment', 'center', 'verticalAlignment', 'base');text(0.5, 0.4, 'Event', 'horizontalAlignment', 'center', 'verticalAlignment', 'base');
  wires:
  Bus Selector3/1 -> Data Type Conversion16/1  "<TSS>"
  Data Type Conversion1/1 -> CanTx1/1
  Data Type Conversion/1 -> CanTx1/2
  Bus Selector5/2 -> Data Type Conversion/1  "<Torque_MCU_Req>"
  Bus Selector2/3 -> CanTx7/3  "<btnY_Input>"
  PostPL_Bus/1 -> Bus Selector/1, Bus Selector1/1, Bus Selector2/1, Bus Selector4/1, Bus Selector5/1, Bus Selector3/1
  Bus Selector3/5 -> Data Type Conversion20/1  "<Operation_Mode>"
  Bus Selector3/4 -> Data Type Conversion19/1  "<Control_Word>"
  Bus Selector3/3 -> Data Type Conversion18/1  "<MCU_NMT_Mode>"
  Bus Selector3/2 -> Data Type Conversion17/1  "<Throttle_Bool>"
  Bus Selector2/2 -> CanTx7/2  "<btnX_Input>"
  Bus Selector2/1 -> CanTx7/1  "<btnRTD_Input>"
  Bus Selector2/8 -> Data Type Conversion13/1  "<LV_Battery_Voltage>"
  Bus Selector5/1 -> Data Type Conversion1/1  "<Throttle_Req>"
  Bus Selector3/6 -> Data Type Conversion21/1  "<Brake_Bool>"
  Bus Selector/1 -> Data Type Conversion4/1  "<Throttle1_Voltage>"
  Bus Selector/2 -> Data Type Conversion2/1  "<Throttle2_Voltage>"
  Bus Selector1/4 -> Data Type Conversion10/1  "<Throttle1_Per>"
  Bus Selector1/5 -> Data Type Conversion9/1  "<Throttle2_Per>"
  Bus Selector1/3 -> Data Type Conversion8/1  "<Brake_Percentage>"
  Bus Selector1/6 -> Data Type Conversion5/1  "<Throttle_Percentage>"
  Data Type Conversion2/1 -> CanTx9/2
  Data Type Conversion4/1 -> CanTx9/1
  Data Type Conversion5/1 -> CanTx6/7
  Data Type Conversion8/1 -> CanTx6/3
  Data Type Conversion9/1 -> CanTx6/6
  Data Type Conversion10/1 -> CanTx6/5
  Data Type Conversion13/1 -> CanTx7/8
  Data Type Conversion16/1 -> CanTx8/1
  Data Type Conversion17/1 -> CanTx8/2
  Data Type Conversion18/1 -> CanTx8/3
  Data Type Conversion19/1 -> CanTx8/4
  Data Type Conversion20/1 -> CanTx8/5
  Data Type Conversion21/1 -> CanTx8/6
  Bus Selector2/4 -> CanTx7/4  "<btnZ_Input>"
  Bus Selector2/7 -> Data Type Conversion12/1  "<Buzzer>"
  Bus Selector4/9 -> Data Type Conversion31/1  "<Shutdown_Error>"
  Memory read/1 -> Data Type Conversion23/1
  Bus Selector4/1 -> Data Type Conversion25/1  "<ECU_Ok>"
  Bus Selector4/2 -> Data Type Conversion27/1  "<AIRLow>"
  Bus Selector4/3 -> Data Type Conversion26/1  "<AIRHigh>"
  Bus Selector4/4 -> Data Type Conversion28/1  "<BPPS_Implausibility>"
  Bus Selector4/5 -> Data Type Conversion11/1  "<Pedal_Sensor_Fail>"
  Bus Selector4/6 -> Data Type Conversion29/1  "<APPS_Implausibility>"
  Bus Selector4/7 -> Data Type Conversion30/1  "<APPS_BP_Implausibility>"
  Bus Selector4/8 -> Data Type Conversion32/1  "<LV_Warning>"
  Bus Selector2/5 -> CanTx7/5  "<PumpFanPower>"
  Data Type Conversion11/1 -> CanTx2/5
  Data Type Conversion12/1 -> CanTx7/7
  Data Type Conversion25/1 -> CanTx2/1
  Data Type Conversion26/1 -> CanTx2/3
  Data Type Conversion27/1 -> CanTx2/2
  Data Type Conversion28/1 -> CanTx2/4
  Data Type Conversion29/1 -> CanTx2/6
  Data Type Conversion30/1 -> CanTx2/7
  Data Type Conversion31/1 -> CanTx2/8
  Data Type Conversion32/1 -> CanTx2/9
  Bus Selector2/6 -> CanTx7/6  "<AccyFanPower>"
  Bus Selector/3 -> Data Type Conversion3/1  "<Brake1_Pressure>"
  Data Type Conversion3/1 -> CanTx9/3
  Bus Selector/4 -> Data Type Conversion6/1  "<Brake2_Pressure>"
  Data Type Conversion6/1 -> CanTx9/4
  Bus Selector1/1 -> Data Type Conversion14/1  "<Brake1_Per>"
  Bus Selector1/2 -> Data Type Conversion7/1  "<Brake2_Per>"
  Data Type Conversion7/1 -> CanTx6/2
  Data Type Conversion14/1 -> CanTx6/1
  Bus Selector2/9 -> Data Type Conversion15/1  "<LV_SOC%>"
  Bus Selector2/10 -> Data Type Conversion22/1  "<Fan_Freq>"
  Data Type Conversion15/1 -> CanTx7/9
  Data Type Conversion22/1 -> CanTx7/10
  Memory read1/1 -> Data Type Conversion24/1
  Ground/1 -> CanTx2/12
  Ground1/1 -> CanTx2/13
  Ground2/1 -> CanTx2/14
  Ground3/1 -> CanTx6/4
  Data Type Conversion23/1 -> CanTx2/11
  Data Type Conversion24/1 -> CanTx2/10

== system TBRe19_ECU_1_WORKING_190718/MainTask ==
  note: Outputs
  note: Convert data to outputs
  note: Data processing
  note: Convert inputs to data
  note: Gather inputs
  note: Overall Functionality:
      | Main vehicle flow diagram
  Comms_And_Data_Acquisition_Layer : Subsystem
  Comms_And_Data_Output_Layer : Subsystem
  Init : Subsystem  mask(System Initialize){}
      mask help: Add code to a systems Initialize function
      settings: CopyFcn=cccopyfcn(gcb)  OpenFcn=ccopenfcn('System Initialize Function')
      mask Help: This block contains text fields to insert custom user code sections at the declaration, execution and exit sections of the systems initialize function.  By placing this block inside a subsytem, the custom user code will appear in that subsystems function.
      mask Display: disp('I()')
  Post_Processing_Layer : Subsystem
  Pre_Processing_Layer : Subsystem
  Task : S-Function  FunctionName=NsiSys_TaskREF  Parameters=task_initialised,task_periodic, task_sampletime,task_name,task_event,task_offset  SFunctionDeploymentMode=off  EnableBusSupport=off  mask(task definition){task_initialised=on, task_periodic=on, task_sampletime=[0.01], task_offset=0.00, task_name=MainTask, task_event=on}
      mask prompts: task_initialised "task initialised"; task_periodic "Is Periodic"; task_sampletime "Task sample time"; task_offset "Task Offset"; task_name "Task name"; task_event "Is event"
      mask help:
      | Permit to provide all parameters associated to a MUXLINK task.
      | Task can be executed periodicaly and/or on event detection.
      | If task is periodic:
      | Task sample time specify the execution period in mS [0.001   6000]
      | Task Offset specify the offset applied to the execution period
      | Task Offset < Task sample time
      mask init:
      | NsiSys_TaskREF_InitializationFcn();
      settings: OpenFcn=NsiSys_Task_OpenFcn();
      mask Callback task_initialised: NsiSys_TaskREF_ApplyFcn(1);
      mask Callback task_periodic: NsiSys_TaskREF_ApplyFcn(2);
      mask Callback task_sampletime: NsiSys_TaskREF_ApplyFcn(3);
      mask Callback task_offset: NsiSys_TaskREF_ApplyFcn(6);
      mask Callback task_name: NsiSys_TaskREF_ApplyFcn(4);
      mask Callback task_event: NsiSys_TaskREF_ApplyFcn(5);
      mask Display: text(0.5, 0.8, 't()', 'horizontalAlignment', 'center', 'verticalAlignment', 'base');text(0.5, 0.2, '/ 10.0ms / 0.0ms /', 'horizontalAlignment', 'center', 'verticalAlignment', 'base');text(0.5, 0.4, 'Event', 'horizontalAlignment', 'center', 'verticalAlignment', 'base');
  Vehicle_Functionality_Layer : Subsystem
  Data_Bus : Outport
  wires:
  Comms_And_Data_Acquisition_Layer/1(DAL_Data) -> Pre_Processing_Layer/1(DAL_Data)
  Pre_Processing_Layer/1(PrePL_Data) -> Vehicle_Functionality_Layer/1(PrePL_Data)
  Vehicle_Functionality_Layer/1(VFL_Data) -> Post_Processing_Layer/1(VFL_Data)
  Post_Processing_Layer/1(PostPL_Data) -> Data_Bus/1, Comms_And_Data_Output_Layer/1(PostPL_Data)

== system TBRe19_ECU_1_WORKING_190718/DiagnosticsCAN/Init ==

== system TBRe19_ECU_1_WORKING_190718/MainTask/Comms_And_Data_Acquisition_Layer ==
  note: CAN_Signals
  note: Overall Functionality:
      | Gather inputs from hardware pins as well as CAN
  BMS_CAN : Subsystem
  Bus Creator : BusCreator  Inputs=2
  Bus Creator1 : BusCreator  Inputs=3
  Hardwired_Inputs_2019 : Subsystem
  MCU_CAN : Subsystem
  SENSOR_CAN : Subsystem
  DAL_Data : Outport
  wires:
  Bus Creator/1 -> DAL_Data/1
  Bus Creator1/1 -> Bus Creator/2  "DAL_CAN"
  Hardwired_Inputs_2019/1(Hardwired_Inputs) -> Bus Creator/1  "DAL_Hardwired"
  MCU_CAN/1(HAL_MCU) -> Bus Creator1/1  "DAL_MCUCAN"
  BMS_CAN/1(BMS_Data) -> Bus Creator1/2  "DAL_BMSCAN"
  SENSOR_CAN/1(Sensor_Data) -> Bus Creator1/3  "DAL_SENSORCAN"

== system TBRe19_ECU_1_WORKING_190718/MainTask/Comms_And_Data_Output_Layer ==
  note: Overall Functionality:
      | Sends outputs from hardware pins as well as to CAN
  PostPL_Data : Inport
  Hardwired_Ouputs : Subsystem
  LEDs : Subsystem
  MCU_CAN : Subsystem
  wires:
  PostPL_Data/1 -> MCU_CAN/1(PostPL_Data), LEDs/1(PostPL_Data), Hardwired_Ouputs/1(PostPL_Data)

== system TBRe19_ECU_1_WORKING_190718/MainTask/Init ==

== system TBRe19_ECU_1_WORKING_190718/MainTask/Post_Processing_Layer ==
  note: Overall Functionality:
      | Post process the results received from the previous layer in order to ensure that all values are within range and plausible for outputs. This includes some minor vehicle funcitonality to set outputs based on demands from VFL.
  VFL_Data : Inport
  Bus Creator1 : BusCreator  Inputs=3
  Dash_LEDs : Subsystem
  Hardwired_Peripherals : Subsystem
  PostPL_Data : Outport
  wires:
  VFL_Data/1 -> Dash_LEDs/1(VFL_Data), Bus Creator1/1, Hardwired_Peripherals/1(VFL_Data)  "VFL_Data"
  Bus Creator1/1 -> PostPL_Data/1
  Hardwired_Peripherals/1(Hardwired_Peripherals) -> Bus Creator1/2  "Hardwired_Peripherals"
  Dash_LEDs/1(LED) -> Bus Creator1/3  "LEDs"

== system TBRe19_ECU_1_WORKING_190718/MainTask/Pre_Processing_Layer ==
  note: Overall Functionality:
      | Pre process the inputs received from the previous layer in order to ensure that all values are within range and plausible. This includes ensuring Motor temperatures are within range, pedal box implausibility, and LV battery voltage monitoring.
  note: Required Changes:
      | Delete signal conversion block if not needed
  DAL_Data : Inport
  Bus Creator : BusCreator  Inputs=5
  Button_Debouncing : Subsystem  mask{DelayLen=5}
      mask prompts: DelayLen "Delay Length"
  LV_Battery : Subsystem
  MCU_Temps : Subsystem
  Pedal_Box : Subsystem
  Signal Conversion : SignalConversion  OverrideOpt=off
  PrePL_Data : Outport
  wires:
  Bus Creator/1 -> PrePL_Data/1
  DAL_Data/1 -> Signal Conversion/1  "HAL_Data"
  Pedal_Box/1(Pedal_Box_Data) -> Bus Creator/3  "Pedal_Box_Data"
  LV_Battery/1(LV_Data) -> Bus Creator/4  "LV_Battery"
  MCU_Temps/1(Temp_Data) -> Bus Creator/2  "MCU_Temps_Data"
  Signal Conversion/1 -> Bus Creator/1, MCU_Temps/1(DAL_Data), Button_Debouncing/1(DAL_Data), LV_Battery/1(DAL_Data), Pedal_Box/1(DAL_In)  "DAL_Data"
  Button_Debouncing/1(Buttons) -> Bus Creator/5  "Buttons"

== system TBRe19_ECU_1_WORKING_190718/MainTask/Vehicle_Functionality_Layer ==
  note: Overall Functionality:
      | Contains vehicle sate machine for RTD and putting VCU in error state, set tractive system startup line.
      | Set Torque values from accel % including traction control and regen
  PrePL_Data : Inport
  Bus Creator : BusCreator  Inputs=3
  Drive_Function : Subsystem
  Vehicle_Operation_Mode : Subsystem
  VFL_Data : Outport
  wires:
  PrePL_Data/1 -> Bus Creator/1, Drive_Function/2(DAL_Data), Vehicle_Operation_Mode/1(PrePL_Data)  "PrePL_Data"
  Vehicle_Operation_Mode/1(VOM_Data) -> Drive_Function/1(Vehicle_Operation_Data), Bus Creator/2  "VOM_Data"
  Bus Creator/1 -> VFL_Data/1
  Drive_Function/1(Drive_Data) -> Bus Creator/3  "Drive_Data"

== system TBRe19_ECU_1_WORKING_190718/MainTask/Comms_And_Data_Acquisition_Layer/BMS_CAN ==
  note: Overall Functionality:
      | Read CAN messages related to BMS
  Bus Creator4 : BusCreator  Inputs=9
  CanRx6 : S-Function  FunctionName=NsiCan_Rx_Ext  Parameters=data_can,channel,msg_name,ident,ident_type,dlc,signals,is_trigger,is_physical,is_canfd,is_rxgw  SFunctionDeploymentMode=off  EnableBusSupport=off  mask(MUXlink Can Rx){data_can=1;HIGH_SPEED;500Kbps;No;C:\Users\Peter\Google_Drive\Year_5\TBRe\03-Design_Files\ECU\ECU-Model\TBRe19_DBC.dbc;0;;;0;HIGH_SPEED;500Kbps;120 Ohm;C:\Users\TBRe-admin\Documents\Database\TBRe19_DBC_190517.dbc;0;;;0;HIGH_SPEED;1000Kbps;120 Ohm;D:\TOOLS\MUXLINK\R2011b\MUXlink\misc\BASE_CAN_MUXLAB4.dbc;0;;;0;HIGH_SPEED;500Kbps;120 Ohm;D:\TOOLS\MUXLINK\R2011b\MUXlink\misc\j1939_adapt.dbc;0;;;0;HIGH_SPEED;1000Kbps;No;D:\TOOLS\MUXLINK\R2011b\MUXlink\misc\BASE_CAN_MUXLAB4.dbc;0;;, channel=1, msg_name=BMS_Feedback_1, ident=0x100, ident_type=STD, dlc=7, signals=Instant_Pack_Voltage;1;0;16;0.100000;0.000000;_;Pack_SOC;1;16;16;1.000000;0.000000;_;Pack_Current;1;32;-16;1.000000;0.000000;_;Acu_Fan;1;48;8;1.000000;0.000000;_, is_trigger=0, is_physical=1, is_canfd=0, is_rxgw=0}
      mask prompts: data_can "data can"; msg_name "msg name"
      mask help: Receive a frame from a CAN channel.
      mask init:
      | NsiCan_Rx_Ext_InitializationFcn();
      settings: OpenFcn=NsiCan_Rx_Ext_OpenFcn();
      mask Help:
      | eval('block=get_param(gcb, ''RTWdata'');')
      | web([docroot '\toolbox\MUXlink\html\blocks/' block.MUXlink_BlockType '.html'])
      mask Callback data_can: NsiCan_Rx_Ext_ApplyFcn(1);
      mask Callback channel: NsiCan_Rx_Ext_ApplyFcn(2);
      mask Callback msg_name: NsiCan_Rx_Ext_ApplyFcn(3);
      mask Callback ident: NsiCan_Rx_Ext_ApplyFcn(4);
      mask Callback ident_type: NsiCan_Rx_Ext_ApplyFcn(5);
      mask Callback dlc: NsiCan_Rx_Ext_ApplyFcn(6);
      mask Callback signals: NsiCan_Rx_Ext_ApplyFcn(7);
      mask Callback is_trigger: NsiCan_Rx_Ext_ApplyFcn(8);
      mask Callback is_physical: NsiCan_Rx_Ext_ApplyFcn(9);
      mask Callback is_canfd: NsiCan_Rx_Ext_ApplyFcn(10);
      mask Callback is_rxgw: NsiCan_Rx_Ext_ApplyFcn(11);
      mask Display: image(imread('nsi.bmp'));text(0.5, 0.3, 'RX_BMS_Feedback_1_CAN1', 'horizontalAlignment', 'center', 'verticalAlignment', 'base');plot([0.05 0.05 0.05 0.05 0.05 0.05 0.05 0.05 0.05 0.05]); port_label('output',1, 'Instant_Pack_Voltage'); port_label('output',2, 'Pack_SOC'); port_label('output',3, 'Pack_Current'); port_label('output',4, 'Acu_Fan'); port_label('output',5, 'Status');
  Data Type Conversion : DataTypeConversion  OutDataTypeStr=int16
  Terminator : Terminator
  UsbTx1 : S-Function  FunctionName=NsiUsb_Tx  Parameters=signame,resolution,offset,unite  SFunctionDeploymentMode=off  EnableBusSupport=off  mask(MUXlink Usb Tx){signame=BMS_Voltage, resolution=1, offset=0, unite=V}
      mask prompts: signame "Signal name ?"; resolution "Resolution ?"; offset "Offset ?"; unite "Unit ?"
      mask help: Transmit a frame on the USB Channel.
      mask init:
      | NsiUsb_Tx_InitializationFcn();
      settings: OpenFcn=NsiUsb_Tx_OpenFcn();
      mask Help:
      | eval('block=get_param(gcb, ''RTWdata'');')
      | web([docroot '\toolbox\MUXlink\html\blocks/' block.MUXlink_BlockType '.html'])
      mask Callback signame: NsiUsb_Tx_ApplyFcn(1);
      mask Callback resolution: NsiUsb_Tx_ApplyFcn(2);
      mask Callback offset: NsiUsb_Tx_ApplyFcn(3);
      mask Callback unite: NsiUsb_Tx_ApplyFcn(4);
      mask Display: image(imread('nsi.bmp'));text(0.5, 0.2, 'USB Tx', 'horizontalAlignment', 'center', 'verticalAlignment', 'base');plot([0.05 0.05 0.05 0.05 0.05 0.05 0.05 0.05 0.05 0.05]);port_label('input',1, 'BMS_Voltage');
  BMS_Data : Outport
  wires:
  CanRx6/5 -> Terminator/1
  CanRx6/3 -> Data Type Conversion/1  "Pack_Current"
  CanRx6/1 -> UsbTx1/1, Bus Creator4/1  "Instant_Pack_Voltage"
  CanRx6/4 -> Bus Creator4/4  "Acc_Fan_Speed"
  Bus Creator4/1 -> BMS_Data/1  "BMS_Data"
  CanRx6/2 -> Bus Creator4/2  "Pack_SOC"
  Data Type Conversion/1 -> Bus Creator4/3  "Pack_Current"

== system TBRe19_ECU_1_WORKING_190718/MainTask/Comms_And_Data_Acquisition_Layer/Hardwired_Inputs_2019 ==
  note: Action:
      | Put the inputs into bus and generate output
  note: Overall Functionality:
      | Get inputs from the physical input pins
  AIRs : Subsystem
  BMS : Subsystem
  Bus Creator : BusCreator  Inputs=18
  Buttons : Subsystem
  FrequentialInput1 : S-Function  FunctionName=NsiIo_FrequencyInput  Parameters=channel,max_freq,is_digital_input,DutyCycle,MUXlabType  SFunctionDeploymentMode=off  EnableBusSupport=off  mask(MUXlink I/O Frequential Input){channel=3, max_freq=10KHZ, is_digital_input=off, DutyCycle=off, MUXlabType=0}
      mask prompts: max_freq "Max Frequency"; is_digital_input "Used as Digital Input"; DutyCycle "Duty Cycle"; MUXlabType "MUXlab Type"
      mask help: Read Frequency from I/O Frequential Input.
      mask init:
      | NsiIo_FrequencyInput_InitializationFcn();
      settings: OpenFcn=NsiIo_FrequencyInput_OpenFcn();
      mask Help:
      | eval('block=get_param(gcb, ''RTWdata'');')
      | web([docroot '\toolbox\MUXlink\html\blocks/' block.MUXlink_BlockType '.html'])
      mask Callback channel: NsiIo_FrequencyInput_ApplyFcn(1);
      mask TypeOptions max_freq: 10KHZ | 100KHZ
      mask Callback max_freq: NsiIo_FrequencyInput_ApplyFcn(2);
      mask Callback is_digital_input: NsiIo_FrequencyInput_ApplyFcn(3);
      mask Callback DutyCycle: NsiIo_FrequencyInput_ApplyFcn(4);
      mask Display: image(imread('nsi.bmp'));text(0.5, 0.2, 'FrequencyInput_3  10KHZ', 'horizontalAlignment', 'center', 'verticalAlignment', 'base');plot([0.05 0.05 0.05 0.05 0.05 0.05 0.05 0.05 0.05 0.05]);port_label('output', 1, 'Freq C3');
  Pedal_Box : Subsystem
  VBat : S-Function  FunctionName=NsiIo_Vbat  SFunctionDeploymentMode=off  EnableBusSupport=off  mask(MUXlink I/O VBat){}
      mask help: Battery Voltage
      mask init:
      | NsiIo_Vbat_InitializationFcn();
      settings: OpenFcn=NsiIo_Vbat_OpenFcn();
      mask Help:
      | eval('block=get_param(gcb, ''RTWdata'');')
      | web([docroot '\toolbox\MUXlink\html\blocks/' block.MUXlink_BlockType '.html'])
      mask Display: image(imread('nsi.bmp'));text(0.5, 0.2, 'I/O VBat', 'horizontalAlignment', 'center', 'verticalAlignment', 'base');plot([0.05 0.05 0.05 0.05 0.05 0.05 0.05 0.05 0.05 0.05]);port_label('output', 1, 'Voltage');
  Hardwired_Inputs : Outport
  wires:
  VBat/1 -> Bus Creator/12  "LV_Battery_Voltage"
  FrequentialInput1/1 -> Bus Creator/13  "Fan_Freq"
  Bus Creator/1 -> Hardwired_Inputs/1
  Pedal_Box/1(Throttle1_Voltage) -> Bus Creator/1
  Pedal_Box/2(Throttle2_Voltage) -> Bus Creator/2
  Pedal_Box/3(Brake_Voltage) -> Bus Creator/3
  Buttons/1(btnRTD_Input) -> Bus Creator/6
  Buttons/2(btnX_Input) -> Bus Creator/7
  Buttons/3(btnY_Input) -> Bus Creator/8
  AIRs/1(AIRLow) -> Bus Creator/14
  AIRs/2(AIRHigh) -> Bus Creator/15
  Pedal_Box/4(Brake1_Pressure) -> Bus Creator/4
  Pedal_Box/5(Brake2_Pressure) -> Bus Creator/5
  Buttons/4(btnZ_Input) -> Bus Creator/9
  Buttons/5(btnPumpFan_Input) -> Bus Creator/10
  Buttons/6(btnAccyFan_Input) -> Bus Creator/11
  BMS/1(BMS_Multi1) -> Bus Creator/16
  BMS/2(BMS_Multi2) -> Bus Creator/17
  BMS/3(BMS_ChargeEnable) -> Bus Creator/18
